simulink model "Assignment_2_Final_Submission"  (R2022b)
settings: Solver=FixedStepAuto  StartTime=0.0  StopTime=10.0  FixedStep=1e-3  RelTol=1e-3  EnableMultiTasking=on
undefined symbols (not defined in the file): A0, A1, D0, D1, D10, D11, D12, D13, D2, D3, D4, D5, D6, D7, D8, D9, magnitude, PTA0, PTA1, PTA2, PTB2, PTB23, PTB3, PTB9, PTC16, PTC17, PTC2, PTC3, PTC4, PTD0, PTD1, PTD2, PTD3
libraries: frdmk64flib x19, etargetslib x8, simulink x2, dspstat3 x1
(part 2 of 2)

== stateflow chart Assignment_2_Final_Submission/Pacing Stateflow ==
  state AOO
    note: This transition ensures we reulate the time spent in each state and pulse at the proper rate. This is the time it takes per one pulse, as determined by the LRL, minus the time spent pulsing.
    note: Atrial mode with no sensing.
        | Constant BPM output.
    state AOO_Charge
      entry:
      PACING_REF_PWM = 100*(ATR_pulseAmplitude/double(5.0));
      pulseTime = 60000/single(LRL);
      % Charging C22
      ATR_PACE_CTRL = false;
      VENT_PACE_CTRL = false;
      PACE_CHARGE_CTRL = true;
      PACE_GND_CTRL = true;
      Z_ATR_CTRL = false;
      Z_VENT_CTRL = false;
      % Discharging C21
      ATR_GND_CTRL = true;
      VENT_GND_CTRL = false;
    state AOO_Discharge
      entry:
      pulseTime = 60000/single(LRL);
      PACE_CHARGE_CTRL = false;
      PACE_GND_CTRL = true;
      ATR_PACE_CTRL = true;
      ATR_GND_CTRL = false;
      Z_ATR_CTRL = false;
      Z_VENT_CTRL = false;
      VENT_GND_CTRL = false;
      VENT_PACE_CTRL = false;
    note: After discharging C22 into the atrium for the
        | desired pulse width, return to the default state
        | to charge C22 and discharge C21.
    AOO.AOO_Charge -> AOO.AOO_Discharge : [after(pulseTime - ATR_pulseWidth, msec)]
    (default) -> AOO.AOO_Charge
    AOO.AOO_Discharge -> AOO.AOO_Charge : [after(ATR_pulseWidth,msec)]
  state VOO
    note: This transition ensures we reulate the time spent in each state and pulse at the proper rate. This is the time it takes per one pulse, as determined by the LRL, minus the time spent pulsing.
    note: Ventricle mode with no sensing.
        | Constant BPM output.
    state VOO_Charge
      entry:
      PACING_REF_PWM = 100*(VENT_pulseAmplitude/double(5.0));
      pulseTime = 60000/single(LRL);
      % Charging C22
      ATR_PACE_CTRL = false;
      VENT_PACE_CTRL = false;
      PACE_CHARGE_CTRL = true;
      PACE_GND_CTRL = true;
      Z_ATR_CTRL = false;
      Z_VENT_CTRL = false;
      % Discharging C21
      ATR_GND_CTRL = false;
      VENT_GND_CTRL = true;
    state VOO_Discharge
      entry:
      pulseTime = 60000/single(LRL);
      PACE_CHARGE_CTRL = false;
      PACE_GND_CTRL = true;
      ATR_PACE_CTRL = false;
      ATR_GND_CTRL = false;
      Z_ATR_CTRL = false;
      Z_VENT_CTRL = false;
      VENT_GND_CTRL = false;
      VENT_PACE_CTRL = true;
    note: After discharging C22 into the ventricle for the
        | desired pulse width, return to the default state
        | to charge C22 and discharge C21.
    VOO.VOO_Charge -> VOO.VOO_Discharge : [after(pulseTime - VENT_pulseWidth, msec)]
    (default) -> VOO.VOO_Charge
    VOO.VOO_Discharge -> VOO.VOO_Charge : [after(VENT_pulseWidth,msec)]
  note: enter state depending on mode set
  state Entry_State
    entry:
    VENT_PACE_CTRL = false;
    ATR_PACE_CTRL = false;
    VENT_GND_CTRL = false;
    ATR_GND_CTRL = false;
    PACE_GND_CTRL = false;
    PACE_CHARGE_CTRL = false;
    FRONTEND_CTRL = true;
    VENT_CMP_REF_PWM = 0;
    ATR_CMP_REF_PWM = 0;
    Z_ATR_CTRL = false;
    Z_VENT_CTRL = false;
    pulseTime = 60000/single(LRL);
    changingPulseTime = (60000/double(changing_LRL));
  state AAI
    pulseTime = 60000/single(LRL);
    note: This state is responsible for charging the pacing circuitry and preparing the system for either sensing or pacing
    note: Moves to the sensing state after the atrial refractory period to monitor atrial activity
    state AAI_Sensing
      entry:
      pulseTime = 60000/single(LRL);
      % Charging C22
      FRONTEND_CTRL = true;
      ATR_CMP_REF_PWM = 53;
      PACING_REF_PWM = 100*(ATR_pulseAmplitude / 5.0);
      VENT_PACE_CTRL = false;
      ATR_PACE_CTRL = false;
      PACE_CHARGE_CTRL = true;
      % Discharging C21
      PACE_GND_CTRL = true;
      ATR_GND_CTRL = true;
      VENT_GND_CTRL = false;
    state AAI_Charge
      entry:
      pulseTime = 60000/single(LRL);
      % Charging C22
      FRONTEND_CTRL = true;
      ATR_CMP_REF_PWM = 53;
      PACING_REF_PWM = 100*(ATR_pulseAmplitude / 5.0);
      VENT_PACE_CTRL = false;
      ATR_PACE_CTRL = false;
      PACE_CHARGE_CTRL = true;
      % Discharging C21
      PACE_GND_CTRL = true;
      ATR_GND_CTRL = true;
      VENT_GND_CTRL = false;
    note: Returns to the charging state if atrial activity is detected
    state AAI_Discharge
      entry:
      pulseTime = 60000/single(LRL);
      PACE_CHARGE_CTRL = false;
      PACE_GND_CTRL = true;
      VENT_PACE_CTRL = false;
      ATR_PACE_CTRL = true;
      ATR_GND_CTRL = false;
      VENT_GND_CTRL = false;
    note: Moves to the discharge state to deliver a pacing pulse after the specified time if no natural atrial signal is detected
    note: after the above calculated wait time, go into the recharge state
    (default) -> AAI.AAI_Charge
    AAI.AAI_Charge -> AAI.AAI_Sensing : after(ARP, msec)
    AAI.AAI_Sensing -> AAI.AAI_Charge [order 1] : [ATR_CMP_DETECT == true]
    AAI.AAI_Discharge -> AAI.AAI_Charge : after(ATR_pulseWidth, msec)
    AAI.AAI_Sensing -> AAI.AAI_Discharge [order 2] : after(pulseTime - single(ARP) - ATR_pulseWidth, msec)
  state VVIR
    note: This state is responsible for charging the pacing circuitry and preparing the system for either sensing or pacing
    note: Moves to the sensing state after the ventricular refractory period to monitor ventricle activity
    state VVI_Charge
      entry:
      % Charging C22
      FRONTEND_CTRL = true;
      VENT_CMP_REF_PWM = 53;
      PACING_REF_PWM = 100*(VENT_pulseAmplitude / 5.0);
      VENT_PACE_CTRL = false;
      ATR_PACE_CTRL = false;
      PACE_CHARGE_CTRL = true;
      % Discharging C21
      PACE_GND_CTRL = true;
      ATR_GND_CTRL = false;
      VENT_GND_CTRL = true;
      changingPulseTime = (60000/double(changing_LRL));
    state VVI_Sensing
      entry:
      % Charging C22
      FRONTEND_CTRL = true;
      VENT_CMP_REF_PWM = 53;
      PACING_REF_PWM = 100*(VENT_pulseAmplitude / 5.0);
      VENT_PACE_CTRL = false;
      ATR_PACE_CTRL = false;
      PACE_CHARGE_CTRL = true;
      % Discharging C21
      PACE_GND_CTRL = true;
      ATR_GND_CTRL = false;
      VENT_GND_CTRL = true;
      changingPulseTime = (60000/double(changing_LRL));
    note: Returns to the charging state if ventricle activity is detected
    state VVI_Discharge
      entry:
      PACE_CHARGE_CTRL = false;
      PACE_GND_CTRL = true;
      VENT_PACE_CTRL = true;
      ATR_PACE_CTRL = false;
      ATR_GND_CTRL = false;
      VENT_GND_CTRL = false;
      changingPulseTime = (60000/double(changing_LRL));
    note: Moves to the discharge state to deliver a pacing pulse after the specified time if no natural ventricular signal is detected
    (default) -> VVIR.VVI_Charge
    VVIR.VVI_Charge -> VVIR.VVI_Sensing : after(VRP, msec)
    VVIR.VVI_Sensing -> VVIR.VVI_Charge [order 1] : [VENT_CMP_DETECT == true]
    VVIR.VVI_Sensing -> VVIR.VVI_Discharge [order 2] : after(changingPulseTime - single(VRP) - VENT_pulseWidth, msec)
    VVIR.VVI_Discharge -> VVIR.VVI_Charge : after(VENT_pulseWidth, msec)
  state VVI
    note: This state is responsible for charging the pacing circuitry and preparing the system for either sensing or pacing
    note: Moves to the sensing state after the ventricular refractory period to monitor ventricle activity
    state VVI_Charge
      entry:
      pulseTime = 60000/single(LRL);
      % Charging C22
      FRONTEND_CTRL = true;
      VENT_CMP_REF_PWM = 53;
      PACING_REF_PWM = 100*(VENT_pulseAmplitude / 5.0);
      VENT_PACE_CTRL = false;
      ATR_PACE_CTRL = false;
      PACE_CHARGE_CTRL = true;
      % Discharging C21
      PACE_GND_CTRL = true;
      ATR_GND_CTRL = false;
      VENT_GND_CTRL = true;
    state VVI_Sensing
      entry:
      pulseTime = 60000/single(LRL);
      % Charging C22
      FRONTEND_CTRL = true;
      VENT_CMP_REF_PWM = 53;
      PACING_REF_PWM = 100*(VENT_pulseAmplitude / 5.0);
      VENT_PACE_CTRL = false;
      ATR_PACE_CTRL = false;
      PACE_CHARGE_CTRL = true;
      % Discharging C21
      PACE_GND_CTRL = true;
      ATR_GND_CTRL = false;
      VENT_GND_CTRL = true;
    note: Returns to the charging state if ventricle activity is detected
    state VVI_Discharge
      entry:
      pulseTime = 60000/single(LRL);
      PACE_CHARGE_CTRL = false;
      PACE_GND_CTRL = true;
      VENT_PACE_CTRL = true;
      ATR_PACE_CTRL = false;
      ATR_GND_CTRL = false;
      VENT_GND_CTRL = false;
    note: Moves to the discharge state to deliver a pacing pulse after the specified time if no natural ventricular signal is detected
    (default) -> VVI.VVI_Charge
    VVI.VVI_Charge -> VVI.VVI_Sensing : after(VRP, msec)
    VVI.VVI_Sensing -> VVI.VVI_Charge [order 1] : [VENT_CMP_DETECT == true]
    VVI.VVI_Discharge -> VVI.VVI_Charge : after(VENT_pulseWidth, msec)
    VVI.VVI_Sensing -> VVI.VVI_Discharge [order 2] : after(pulseTime - single(VRP) - VENT_pulseWidth, msec)
  state AAIR
    note: This state is responsible for charging the pacing circuitry and preparing the system for either sensing or pacing
    note: Moves to the sensing state after the atrial refractory period to monitor atrial activity
    state AAI_Sensing
      entry:
      % Charging C22
      FRONTEND_CTRL = true;
      ATR_CMP_REF_PWM = 53;
      PACING_REF_PWM = 100*(ATR_pulseAmplitude / 5.0);
      VENT_PACE_CTRL = false;
      ATR_PACE_CTRL = false;
      PACE_CHARGE_CTRL = true;
      % Discharging C21
      PACE_GND_CTRL = true;
      ATR_GND_CTRL = true;
      VENT_GND_CTRL = false;
      changingPulseTime = (60000/double(changing_LRL));
    state AAI_Charge
      entry:
      % Charging C22
      FRONTEND_CTRL = true;
      ATR_CMP_REF_PWM = 53;
      PACING_REF_PWM = 100*(ATR_pulseAmplitude / 5.0);
      VENT_PACE_CTRL = false;
      ATR_PACE_CTRL = false;
      PACE_CHARGE_CTRL = true;
      % Discharging C21
      PACE_GND_CTRL = true;
      ATR_GND_CTRL = true;
      VENT_GND_CTRL = false;
      changingPulseTime = (60000/double(changing_LRL));
    note: Returns to the charging state if atrial activity is detected
    state AAI_Discharge
      entry:
      PACE_CHARGE_CTRL = false;
      PACE_GND_CTRL = true;
      VENT_PACE_CTRL = false;
      ATR_PACE_CTRL = true;
      ATR_GND_CTRL = false;
      VENT_GND_CTRL = false;
      changingPulseTime = (60000/double(changing_LRL));
    note: Moves to the discharge state to deliver a pacing pulse after the specified time if no natural atrial signal is detected
    note: after the above calculated wait time, go into the recharge state
    (default) -> AAIR.AAI_Charge
    AAIR.AAI_Charge -> AAIR.AAI_Sensing : after(ARP, msec)
    AAIR.AAI_Sensing -> AAIR.AAI_Charge [order 1] : [ATR_CMP_DETECT == true]
    AAIR.AAI_Discharge -> AAIR.AAI_Charge : after(ATR_pulseWidth, msec)
    AAIR.AAI_Sensing -> AAIR.AAI_Discharge [order 2] : after(changingPulseTime - single(ARP) - ATR_pulseWidth, msec)
  state VOOR
    note: This transition ensures we reulate the time spent in each state and pulse at the proper rate. This is the time it takes per one pulse, as determined by the LRL, minus the time spent pulsing.
    note: Ventricle mode with no sensing.
        | Constant BPM output.
    state VOO_Charge
      entry:
      PACING_REF_PWM = 100*(VENT_pulseAmplitude/double(5.0));
      % Charging C22
      ATR_PACE_CTRL = false;
      VENT_PACE_CTRL = false;
      PACE_CHARGE_CTRL = true;
      PACE_GND_CTRL = true;
      Z_ATR_CTRL = false;
      Z_VENT_CTRL = false;
      % Discharging C21
      ATR_GND_CTRL = false;
      VENT_GND_CTRL = true;
      changingPulseTime = (60000/double(changing_LRL));
    state VOO_Discharge
      entry:
      PACE_CHARGE_CTRL = false;
      PACE_GND_CTRL = true;
      ATR_PACE_CTRL = false;
      ATR_GND_CTRL = false;
      Z_ATR_CTRL = false;
      Z_VENT_CTRL = false;
      VENT_GND_CTRL = false;
      VENT_PACE_CTRL = true;
      changingPulseTime = (60000/double(changing_LRL));
    note: After discharging C22 into the ventricle for the
        | desired pulse width, return to the default state
        | to charge C22 and discharge C21.
    VOOR.VOO_Charge -> VOOR.VOO_Discharge : [after(changingPulseTime - VENT_pulseWidth, msec)]
    (default) -> VOOR.VOO_Charge
    VOOR.VOO_Discharge -> VOOR.VOO_Charge : [after(VENT_pulseWidth,msec)]
  state AOOR
    note: This transition ensures we reulate the time spent in each state and pulse at the proper rate. This is the time it takes per one pulse, as determined by the LRL, minus the time spent pulsing.
    note: Atrial mode with no sensing.
        | Constant BPM output.
    state AOO_Charge
      entry:
      PACING_REF_PWM = 100*(ATR_pulseAmplitude/double(5.0));
      % Charging C22
      ATR_PACE_CTRL = false;
      VENT_PACE_CTRL = false;
      PACE_CHARGE_CTRL = true;
      PACE_GND_CTRL = true;
      Z_ATR_CTRL = false;
      Z_VENT_CTRL = false;
      % Discharging C21
      ATR_GND_CTRL = true;
      VENT_GND_CTRL = false;
      changingPulseTime = (60000/double(changing_LRL));
    state AOO_Discharge
      entry:
      PACE_CHARGE_CTRL = false;
      PACE_GND_CTRL = true;
      ATR_PACE_CTRL = true;
      ATR_GND_CTRL = false;
      Z_ATR_CTRL = false;
      Z_VENT_CTRL = false;
      VENT_GND_CTRL = false;
      VENT_PACE_CTRL = false;
      changingPulseTime = (60000/double(changing_LRL));
    note: After discharging C22 into the atrium for the
        | desired pulse width, return to the default state
        | to charge C22 and discharge C21.
    AOOR.AOO_Charge -> AOOR.AOO_Discharge : [after(changingPulseTime - ATR_pulseWidth, msec)]
    (default) -> AOOR.AOO_Charge
    AOOR.AOO_Discharge -> AOOR.AOO_Charge : [after(ATR_pulseWidth,msec)]
  AOO -> Entry_State : [mode ~= 1]
  Entry_State -> AOO [order 1] : [mode == 1]
  Entry_State -> VOO [order 2] : [mode == 2]
  VOO -> Entry_State : [mode ~= 2]
  (default) -> Entry_State
  Entry_State -> AAI [order 4] : [mode == 3]
  VVIR -> Entry_State : [mode ~= 8]
  Entry_State -> VVIR [order 8] : [mode == 8]
  AAI -> Entry_State : [mode ~= 3]
  Entry_State -> VVI [order 3] : [mode == 4]
  AAIR -> Entry_State : [mode ~= 7]
  VVI -> Entry_State : [mode ~= 4]
  Entry_State -> AAIR [order 7] : [mode == 7]
  VOOR -> Entry_State : [mode ~= 6]
  Entry_State -> VOOR [order 6] : [mode == 6]
  AOOR -> Entry_State : [mode ~= 5]
  Entry_State -> AOOR [order 5] : [mode == 5]
  data: changing_LRL input double; mode input uint8; ATR_pulseWidth input single; VENT_pulseWidth input single; VRP input uint16; ARP input uint16; LRL input uint8; VENT_pulseAmplitude input; ATR_pulseAmplitude input; ATR_CMP_DETECT input; VENT_CMP_DETECT input boolean; Z_VENT_CTRL output boolean; ATR_PACE_CTRL output boolean; PACE_CHARGE_CTRL output boolean; PACE_GND_CTRL output boolean; VENT_PACE_CTRL output boolean; VENT_GND_CTRL output boolean; ATR_GND_CTRL output boolean; Z_ATR_CTRL output boolean; FRONTEND_CTRL output; PACING_REF_PWM output; VENT_CMP_REF_PWM output; ATR_CMP_REF_PWM output; pulseTime local single; changingPulseTime local double

== stateflow chart Assignment_2_Final_Submission/Rate Adaptation/Chart ==
  state Init
    entry:
    adaptedRate = double(LRL);
  state Slope_Calculation
    %Calculates slope and desired target depending on input activity
    entry:
    slope = 0.75 * double(responseFactor);
    target = single(LRL) + single(slope)*single(Activity - activityThreshold);
    %Check Min and Max
    if (target > MSR)
    target = single(MSR);
    end
    if (target > URL)
    target = single(URL);
    end
    if (target < LRL)
    target = single(LRL);
    end
  state Rate_Calculation
    %Calculates steps to increment and decrement per cycle in ms
    entry:
    stepReaction = double(MSR - LRL)/(double(reactionTime)*1000);
    stepRecovery = double(MSR - LRL)/(double(recoveryTime)*60000);
    %Increases or decreases rate by min step
    %Multiplying by 100 due to 100msec delay
    if adaptedRate < target
    adaptedRate = double(adaptedRate + double(100)*stepReaction);
    end
    if adaptedRate > target
    adaptedRate = double(adaptedRate - double(100)*stepRecovery);
    end
    if (adaptedRate > URL)
    adaptedRate = double(URL);
    end
    if (adaptedRate < LRL)
    adaptedRate = double(LRL);
    end
  (default) -> Init
  Init -> Slope_Calculation : [true]
  Slope_Calculation -> Rate_Calculation : after(1, msec)
  Rate_Calculation -> Slope_Calculation : after(100, msec)
  data: Activity input uint8; LRL input uint8; adaptedRate output double; URL input uint8; MSR input uint8; activityThreshold input uint8; responseFactor input uint8; reactionTime input uint8; recoveryTime input uint8; slope local double; target local; stepReaction local double; stepRecovery local double

== stateflow chart Assignment_2_Final_Submission/Chart1 ==
  state Intro
    entry:
    Trigger = false;
  state Trigger
    entry:
    Trigger = true;
  (default) -> Intro
  Intro -> Trigger : after(20,msec)
  Trigger -> Intro
  data: Trigger output
